simulink model "Question3_1"  (R2017b)
settings: Solver=VariableStepDiscrete  StartTime=0.0  StopTime=2.0  MaxStep=1e-4  RelTol=1e-3
libraries: powerlib x19
settings Model: Creator=SiF  LastModifiedBy=SiF

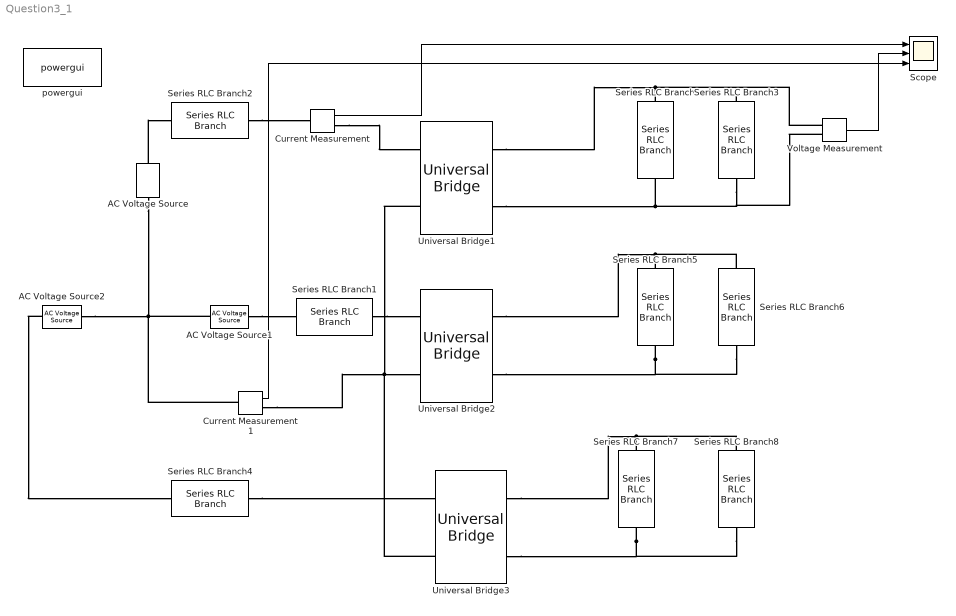
== system Question3_1 ==
  AC Voltage Source : powerlib/Electrical Sources/AC Voltage Source  Amplitude=325.26  Phase=0  Frequency=50  SampleTime=1e-6  Measurements=None  BusType=swing  Pref=10e3  Qref=0  Qmin=-inf  Qmax=+inf
  AC Voltage Source1 : powerlib/Electrical Sources/AC Voltage Source  Amplitude=325.26  Phase=120  Frequency=50  SampleTime=1e-6  Measurements=None  BusType=swing  Pref=10e3  Qref=0  Qmin=-inf  Qmax=+inf
  AC Voltage Source2 : powerlib/Electrical Sources/AC Voltage Source  Amplitude=325.26  Phase=240  Frequency=50  SampleTime=1e-6  Measurements=None  BusType=swing  Pref=10e3  Qref=0  Qmin=-inf  Qmax=+inf
  Current Measurement : powerlib/Measurements/Current Measurement  PhasorSimulation=off  OutputType=Complex  PSBequivalent=0
  Current Measurement1 : powerlib/Measurements/Current Measurement  PhasorSimulation=off  OutputType=Complex  PSBequivalent=0
  Scope : Scope  NumInputPorts=3
  Series RLC Branch : powerlib/Elements/Series RLC Branch  LConnTagsString=__new0  RConnTagsString=__new0  BranchType=R  Resistance=200  Inductance=1  SetiL0=off  InitialCurrent=0  Capacitance=3.7e-7  Setx0=off  InitialVoltage=0  Measurements=None
  Series RLC Branch1 : powerlib/Elements/Series RLC Branch  LConnTagsString=__new0  RConnTagsString=__new0  BranchType=L  Resistance=200  Inductance=600e-6  SetiL0=off  InitialCurrent=0  Capacitance=3.7e-7  Setx0=off  InitialVoltage=0  Measurements=None
  Series RLC Branch2 : powerlib/Elements/Series RLC Branch  LConnTagsString=__new0  RConnTagsString=__new0  BranchType=L  Resistance=200  Inductance=600e-6  SetiL0=off  InitialCurrent=0  Capacitance=3.7e-7  Setx0=off  InitialVoltage=0  Measurements=None
  Series RLC Branch3 : powerlib/Elements/Series RLC Branch  LConnTagsString=__new0  RConnTagsString=__new0  BranchType=C  Resistance=25  Inductance=1  SetiL0=off  InitialCurrent=0  Capacitance=470e-6  Setx0=off  InitialVoltage=0  Measurements=None
  Series RLC Branch4 : powerlib/Elements/Series RLC Branch  LConnTagsString=__new0  RConnTagsString=__new0  BranchType=L  Resistance=200  Inductance=600e-6  SetiL0=off  InitialCurrent=0  Capacitance=3.7e-7  Setx0=off  InitialVoltage=0  Measurements=None
  Series RLC Branch5 : powerlib/Elements/Series RLC Branch  LConnTagsString=__new0  RConnTagsString=__new0  BranchType=R  Resistance=200  Inductance=1  SetiL0=off  InitialCurrent=0  Capacitance=3.7e-7  Setx0=off  InitialVoltage=0  Measurements=None
  Series RLC Branch6 : powerlib/Elements/Series RLC Branch  LConnTagsString=__new0  RConnTagsString=__new0  BranchType=C  Resistance=25  Inductance=1  SetiL0=off  InitialCurrent=0  Capacitance=470e-6  Setx0=off  InitialVoltage=0  Measurements=None
  Series RLC Branch7 : powerlib/Elements/Series RLC Branch  LConnTagsString=__new0  RConnTagsString=__new0  BranchType=R  Resistance=200  Inductance=1  SetiL0=off  InitialCurrent=0  Capacitance=3.7e-7  Setx0=off  InitialVoltage=0  Measurements=None
  Series RLC Branch8 : powerlib/Elements/Series RLC Branch  LConnTagsString=__new0  RConnTagsString=__new0  BranchType=C  Resistance=25  Inductance=1  SetiL0=off  InitialCurrent=0  Capacitance=470e-6  Setx0=off  InitialVoltage=0  Measurements=None
  Universal Bridge1 : powerlib/Power Electronics/Universal Bridge  Arms=2  SnubberResistance=1e5  SnubberCapacitance=inf  Device=Diodes  Ron=1e-3  Lon=0  ForwardVoltages="[  0  0  ]"  ForwardVoltage=0  GTOparameters=[ 10e-6 , 20e-6 ]  IGBTparameters=[ 1e-6 , 2e-6 ]  Measurements=None  Measurements_2=None  converterType=Rectifier
  Universal Bridge2 : powerlib/Power Electronics/Universal Bridge  Arms=2  SnubberResistance=1e5  SnubberCapacitance=inf  Device=Diodes  Ron=1e-3  Lon=0  ForwardVoltages="[  0  0  ]"  ForwardVoltage=0  GTOparameters=[ 10e-6 , 20e-6 ]  IGBTparameters=[ 1e-6 , 2e-6 ]  Measurements=None  Measurements_2=None  converterType=Rectifier
  Universal Bridge3 : powerlib/Power Electronics/Universal Bridge  Arms=2  SnubberResistance=1e5  SnubberCapacitance=inf  Device=Diodes  Ron=1e-3  Lon=0  ForwardVoltages="[  0  0  ]"  ForwardVoltage=0  GTOparameters=[ 10e-6 , 20e-6 ]  IGBTparameters=[ 1e-6 , 2e-6 ]  Measurements=None  Measurements_2=None  converterType=Rectifier
  Voltage Measurement : powerlib/Measurements/Voltage Measurement  PhasorSimulation=off  OutputType=Complex  PSBequivalent=0
  powergui : powerlib/powergui  Priority=1  SimulationMode=Discrete  SampleTime=1e-6  frequency=60  Iterations=50  frequencyindice=50  Pbase=100e6  ErrMax=1e-4  UnitsV=kV  UnitsW=MW  buscounter=0  FunctionMessages=off  echomessages=off  EnableUseOfTLC=off  CurrentSourceSwitches=off  DisableSnubberDevices=off  DisableRonSwitches=off  DisableVfSwitches=off  DisplayEquations=off  SolverType=Tustin/Backward Euler (TBE)  Interpol=off  ExternalGateDelay=off  methode=off  Ts=100  x0status=blocks  SPID=on  SwTol=0  HookPort=off  RestoreLinks=warning  ResistiveCurrentMeasurement=off  Frange=[0:2:500]  Ylog=off  Xlog=on  ShowGrid=off  save=off  variable=ZData  structure=ScopeData  ZoomFFT=off  StartTime=0.8  cycles=5  DisplayStyle=1  fundamental=50  FreqAxis=off  MaxFrequency=1000  frequencyindicesteady=1  RmsSteady=1  display=off
  wires:
  Current Measurement/1 -> Scope/1
  Voltage Measurement/1 -> Scope/2
  Current Measurement1/1 -> Scope/3
  connections:
  Series RLC Branch/LConn1 -- Voltage Measurement/LConn1 -- Series RLC Branch3/LConn1 -- Universal Bridge1/RConn1
  Universal Bridge1/RConn2 -- Voltage Measurement/LConn2 -- Series RLC Branch3/RConn1 -- Series RLC Branch/RConn1
  Universal Bridge2/RConn1 -- Series RLC Branch6/LConn1 -- Series RLC Branch5/LConn1
  Series RLC Branch5/RConn1 -- Series RLC Branch6/RConn1 -- Universal Bridge2/RConn2
  Universal Bridge3/RConn1 -- Series RLC Branch8/LConn1 -- Series RLC Branch7/LConn1
  Series RLC Branch7/RConn1 -- Series RLC Branch8/RConn1 -- Universal Bridge3/RConn2
  Current Measurement/RConn1 -- Universal Bridge1/LConn1
  AC Voltage Source/LConn1 -- AC Voltage Source1/LConn1 -- Current Measurement1/LConn1 -- AC Voltage Source2/LConn1
  Series RLC Branch1/LConn1 -- Universal Bridge2/LConn1
  Series RLC Branch4/LConn1 -- Universal Bridge3/LConn1
  Series RLC Branch2/LConn1 -- Current Measurement/LConn1
  Universal Bridge1/LConn2 -- Current Measurement1/RConn1 -- Universal Bridge3/LConn2 -- Universal Bridge2/LConn2
  AC Voltage Source/RConn1 -- Series RLC Branch2/RConn1
  AC Voltage Source1/RConn1 -- Series RLC Branch1/RConn1
  AC Voltage Source2/RConn1 -- Series RLC Branch4/RConn1
